simulink model "diag_bloqu"  (R2022a)
settings: Solver=VariableStepAuto  StartTime=0.0  StopTime=30  RelTol=1e-3
settings Model: Creator=Adriana  LastModifiedBy=Adriana

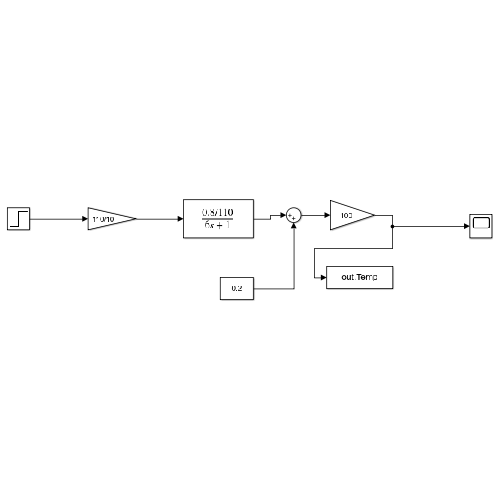
[thumbnail: Simulink's stored preview of the top-level diagram]
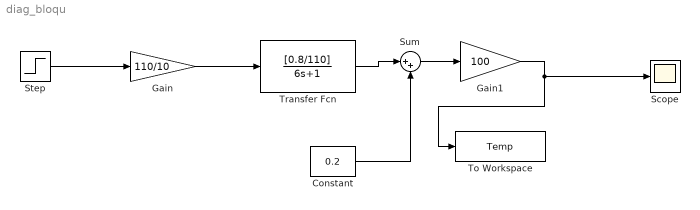
== system diag_bloqu ==
  Constant : Constant  Value=0.2
  Gain : Gain  Gain=110/10
  Gain1 : Gain  Gain=100
  Scope : Scope
  Step : Step  Time=0  After=10  SampleTime=0
  Sum : Sum  Inputs=|++
  To Workspace : ToWorkspace  VariableName=Temp  SaveFormat=Timeseries  SampleTime=-1
  Transfer Fcn : TransferFcn  Numerator=[0.8/110]  Denominator=[6 1]
  wires:
  Step/1 -> Gain/1
  Gain/1 -> Transfer Fcn/1
  Transfer Fcn/1 -> Sum/1
  Constant/1 -> Sum/2
  Sum/1 -> Gain1/1
  Gain1/1 -> Scope/1, To Workspace/1
